simulink model "A3ii"  (R2019b)
settings: Solver=VariableStepAuto  StartTime=0.0  StopTime=0.8  RelTol=1e-3
settings Model: Creator=mluser  LastModifiedBy=KK

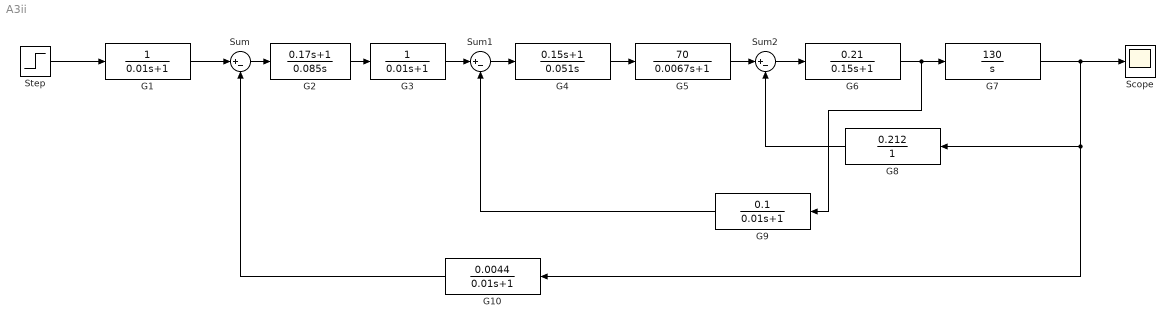
== system A3ii ==
  G1 : TransferFcn  Denominator=[0.01 1]
  G10 : TransferFcn  Numerator=[0.0044]  Denominator=[0.01 1]
  G2 : TransferFcn  Numerator=[0.17 1]  Denominator=[0.085 0]
  G3 : TransferFcn  Denominator=[0.01 1]
  G4 : TransferFcn  Numerator=[0.15 1]  Denominator=[0.051 0]
  G5 : TransferFcn  Numerator=[70]  Denominator=[0.0067 1]
  G6 : TransferFcn  Numerator=[0.21]  Denominator=[0.15 1]
  G7 : TransferFcn  Numerator=[130]  Denominator=[1 0]
  G8 : TransferFcn  Numerator=[0.212]  Denominator=[1]
  G9 : TransferFcn  Numerator=[0.1]  Denominator=[0.01 1]
  Scope : Scope
  Step : Step  Before=1  After=0  SampleTime=0
  Sum : Sum  Inputs=|+-
  Sum1 : Sum  Inputs=|+-
  Sum2 : Sum  Inputs=|+-
  wires:
  G1/1 -> Sum/1
  Sum/1 -> G2/1
  G2/1 -> G3/1
  Sum1/1 -> G4/1
  G3/1 -> Sum1/1
  G4/1 -> G5/1
  G6/1 -> G9/1, G7/1
  G7/1 -> G10/1, G8/1, Scope/1
  G9/1 -> Sum1/2
  G10/1 -> Sum/2
  G8/1 -> Sum2/2
  Sum2/1 -> G6/1
  G5/1 -> Sum2/1
  Step/1 -> G1/1
